simulink subsystem "MSD_ode"  (R2022a)
settings: Solver=VariableStepAuto  StartTime=0.0  StopTime=10.0  RelTol=1e-3
values from neighbouring files (symbols this model uses):
  b = SIM.b    [KalmanTesting_Mechanical.m]    (also in KalmanTesting_Mechanical_DataGeneration.m; KalmanTesting_Mechanical_InputQ_Sine.m; KalmanTesting_Mechanical_InputQ_Step.m; KalmanTesting_Mechanical_InputQ_Step_DataGen.m)
  C = [1 1 1 1]    [KalmanTesting_Mechanical.m]    (also in KalmanTesting_Mechanical_DataGeneration.m = [0 0 0 1]; KalmanTesting_Mechanical_InputQ_Sine.m = [0 0 0 1]; KalmanTesting_Mechanical_InputQ_Step.m = [1 0 0 0]; KalmanTesting_Mechanical_InputQ_Step_DataGen.m = [0 0 0 1])
  k1 = SIM.k1    [KalmanTesting_Mechanical.m]    (also in KalmanTesting_Mechanical_DataGeneration.m; KalmanTesting_Mechanical_InputQ_Sine.m; KalmanTesting_Mechanical_InputQ_Step.m; KalmanTesting_Mechanical_InputQ_Step_DataGen.m)
  k2 = SIM.k2    [KalmanTesting_Mechanical.m]    (also in KalmanTesting_Mechanical_DataGeneration.m; KalmanTesting_Mechanical_InputQ_Sine.m; KalmanTesting_Mechanical_InputQ_Step.m; KalmanTesting_Mechanical_InputQ_Step_DataGen.m)
  m1 = SIM.m1    [KalmanTesting_Mechanical.m]    (also in KalmanTesting_Mechanical_DataGeneration.m; KalmanTesting_Mechanical_InputQ_Sine.m; KalmanTesting_Mechanical_InputQ_Step.m; KalmanTesting_Mechanical_InputQ_Step_DataGen.m)
  m2 = SIM.m2    [KalmanTesting_Mechanical.m]    (also in KalmanTesting_Mechanical_DataGeneration.m; KalmanTesting_Mechanical_InputQ_Sine.m; KalmanTesting_Mechanical_InputQ_Step.m; KalmanTesting_Mechanical_InputQ_Step_DataGen.m)
undefined symbols (not defined in the file or in its folder): x0
settings Model: Creator=tyevans  LastModifiedBy=tyevans

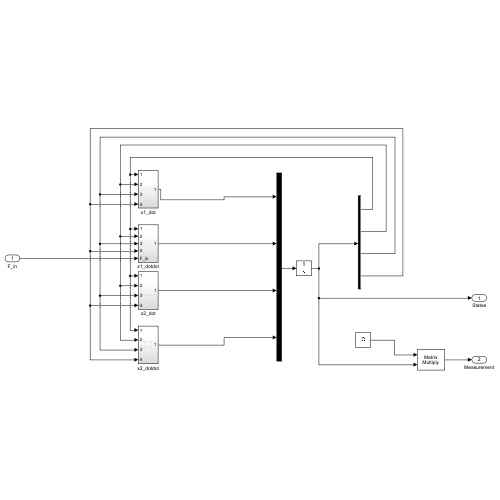
[thumbnail: Simulink's stored preview of the top-level diagram]
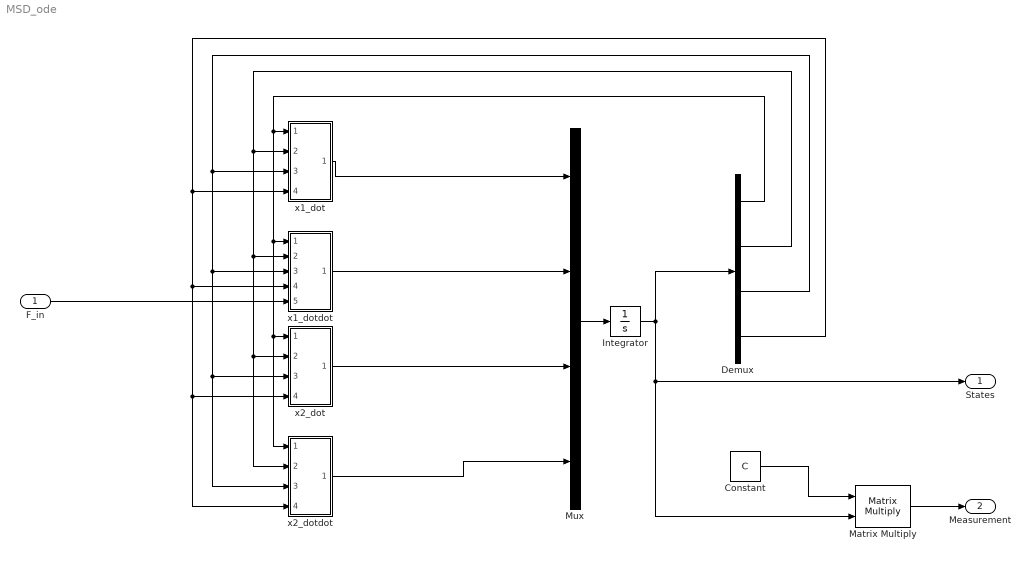
== system MSD_ode ==
  F_in : Inport
  Constant : Constant  Value=C  VectorParams1D=off
  Demux : Demux
  Integrator : Integrator  InitialCondition=x0
  Matrix Multiply : Product  Multiplication=Matrix(*)
  Mux : Mux
  x1_dot : Subsystem
  x1_dotdot : Subsystem
  x2_dot : Subsystem
  x2_dotdot : Subsystem
  States : Outport
  Measurement : Outport  Port=2
  wires:
  Demux/4 -> x1_dot/4(In4), x2_dot/4(In4), x2_dotdot/4(In4), x1_dotdot/4(In4)
  Demux/1 -> x1_dot/1(In1), x1_dotdot/1(In1), x2_dot/1(In1), x2_dotdot/1(In1)
  x2_dot/1(Out1) -> Mux/3
  x2_dotdot/1(Out1) -> Mux/4
  x1_dotdot/1(Out1) -> Mux/2
  Demux/2 -> x1_dot/2(In2), x1_dotdot/2(In2), x2_dot/2(In2), x2_dotdot/2(In2)
  x1_dot/1(Out1) -> Mux/1
  Integrator/1 -> Demux/1, States/1, Matrix Multiply/2
  Demux/3 -> x1_dot/3(In3), x2_dot/3(In3), x2_dotdot/3(In3), x1_dotdot/3(In3)
  Mux/1 -> Integrator/1
  F_in/1 -> x1_dotdot/5(F_in)
  Matrix Multiply/1 -> Measurement/1
  Constant/1 -> Matrix Multiply/1

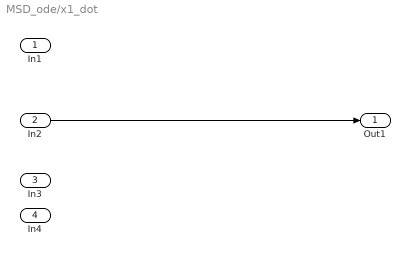
== system MSD_ode/x1_dot ==
  In1 : Inport
  In2 : Inport  Port=2
  In3 : Inport  Port=3
  In4 : Inport  Port=4
  Out1 : Outport
  wires:
  In2/1 -> Out1/1

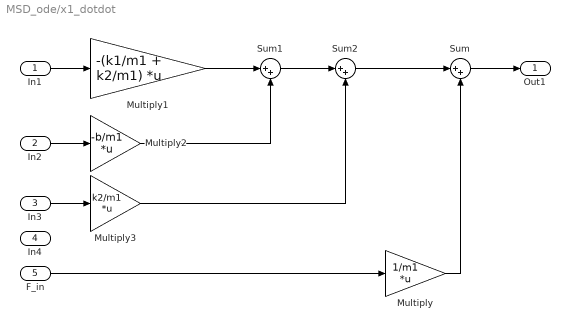
== system MSD_ode/x1_dotdot ==
  In1 : Inport
  In2 : Inport  Port=2
  In3 : Inport  Port=3
  In4 : Inport  Port=4
  F_in : Inport  Port=5
  Multiply : Gain  Gain=1/m1  Multiplication=Matrix(K*u)
  Multiply1 : Gain  Gain=-(k1/m1 + k2/m1)  Multiplication=Matrix(K*u)
  Multiply2 : Gain  Gain=-b/m1  Multiplication=Matrix(K*u)
  Multiply3 : Gain  Gain=k2/m1  Multiplication=Matrix(K*u)
  Sum : Sum  Inputs=|++
  Sum1 : Sum  Inputs=|++
  Sum2 : Sum  Inputs=|++
  Out1 : Outport
  wires:
  Multiply3/1 -> Sum2/2
  In3/1 -> Multiply3/1
  Multiply2/1 -> Sum1/2
  In2/1 -> Multiply2/1
  In1/1 -> Multiply1/1
  Sum/1 -> Out1/1
  Sum2/1 -> Sum/1
  Sum1/1 -> Sum2/1
  Multiply1/1 -> Sum1/1
  Multiply/1 -> Sum/2
  F_in/1 -> Multiply/1

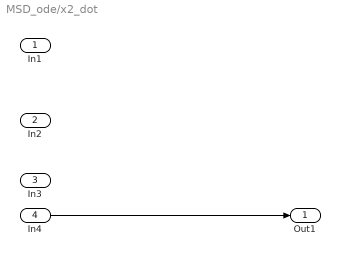
== system MSD_ode/x2_dot ==
  In1 : Inport
  In2 : Inport  Port=2
  In3 : Inport  Port=3
  In4 : Inport  Port=4
  Out1 : Outport
  wires:
  In4/1 -> Out1/1

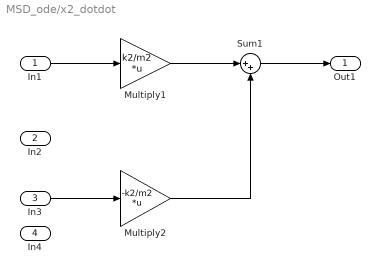
== system MSD_ode/x2_dotdot ==
  In1 : Inport
  In2 : Inport  Port=2
  In3 : Inport  Port=3
  In4 : Inport  Port=4
  Multiply1 : Gain  Gain=k2/m2  Multiplication=Matrix(K*u)
  Multiply2 : Gain  Gain=-k2/m2  Multiplication=Matrix(K*u)
  Sum1 : Sum  Inputs=|++
  Out1 : Outport
  wires:
  Sum1/1 -> Out1/1
  Multiply1/1 -> Sum1/1
  In1/1 -> Multiply1/1
  In3/1 -> Multiply2/1
  Multiply2/1 -> Sum1/2
